simulink model "task3"  (R2023b)
settings: Solver=FixedStepDiscrete  StartTime=0.0  StopTime=10.0  FixedStep=5e-5  RelTol=1e-3
PreLoadFcn:
  | Simulink.defineIntEnumType('windowCommand', {'Off','Speed1','Speed2','Speed3'},[0,1,2,3])
settings Model: Creator=kz1nz0  LastModifiedBy=Zuzia

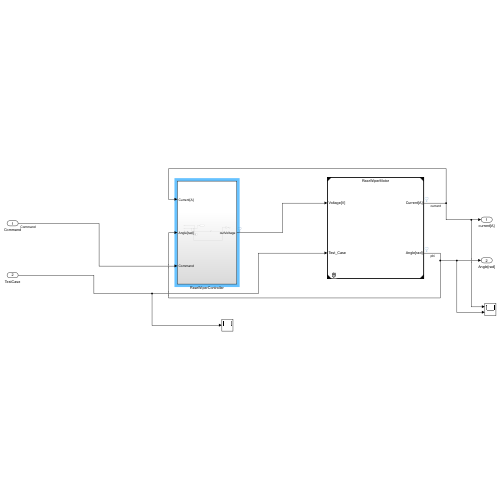
[thumbnail: Simulink's stored preview of the top-level diagram]
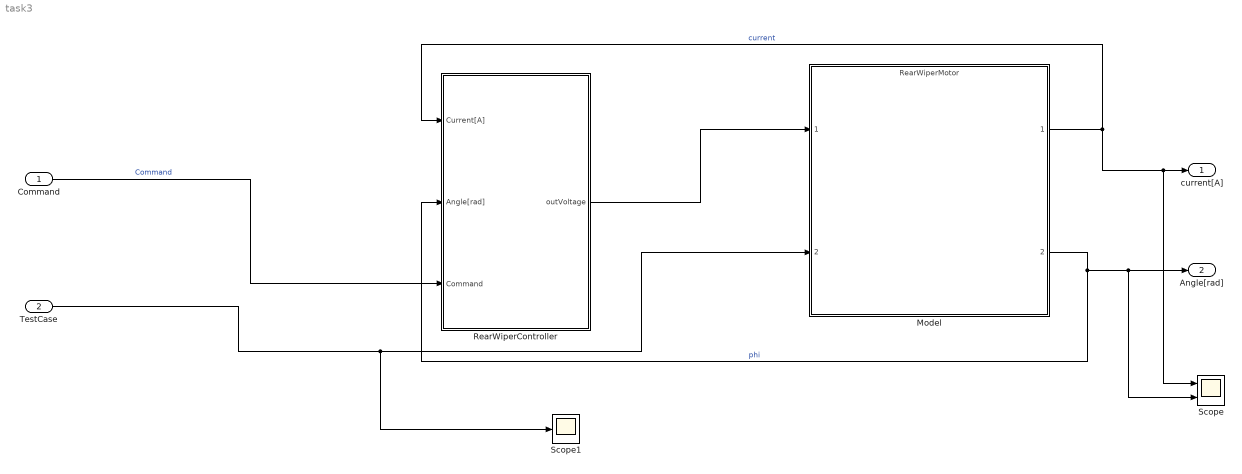
== system task3 ==
  Command : Inport  OutDataTypeStr=Enum: windowCommand
  TestCase : Inport  Port=2  OutDataTypeStr=int8
  Model : ModelReference  ModelNameDialog=RearWiperMotor.slxp  ModelReferenceVersion=19.15  CopyOfModelProtected=on
  RearWiperController : Subsystem
  Scope : Scope  NumInputPorts=2
  Scope1 : Scope
  current[A] : Outport
  Angle[rad] : Outport  Port=2
  wires:
  Command/1 -> RearWiperController/3(Command)  "Command"
  TestCase/1 -> Scope1/1, Model/2
  Model/1 -> Scope/1, current[A]/1, RearWiperController/1(Current[A])  "current"
  Model/2 -> RearWiperController/2(Angle[rad]), Scope/2, Angle[rad]/1  "phi"
  RearWiperController/1(outVoltage) -> Model/1

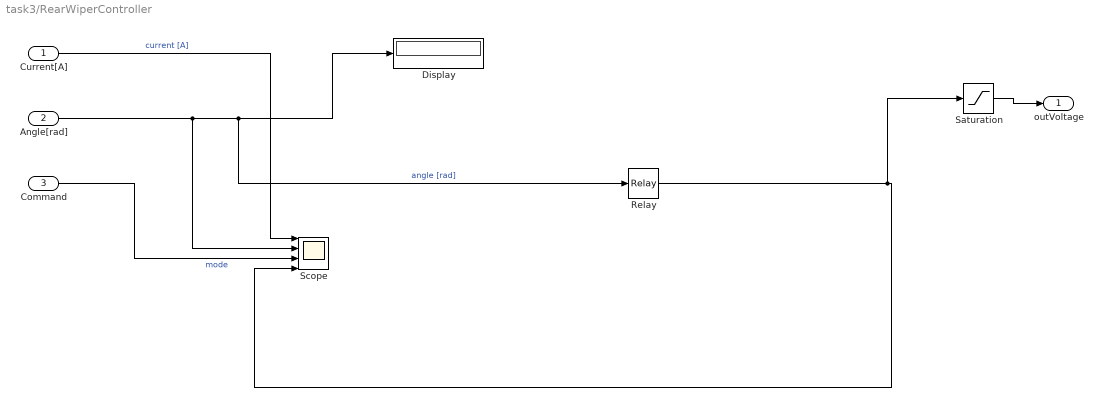
== system task3/RearWiperController ==
  Current[A] : Inport
  Angle[rad] : Inport  Port=2
  Command : Inport  Port=3  OutDataTypeStr=Enum: windowCommand
  Display : Display
  Relay : Relay  OnSwitchValue=2.7  OffSwitchValue=0  OnOutputValue=-5  OffOutputValue=5
  Saturation : Saturate  UpperLimit=12  LowerLimit=-12
  Scope : Scope  NumInputPorts=4
  outVoltage : Outport
  wires:
  Command/1 -> Scope/3  "mode"
  Angle[rad]/1 -> Scope/2, Relay/1, Display/1  "angle [rad]"
  Current[A]/1 -> Scope/1  "current [A]"
  Relay/1 -> Saturation/1, Scope/4
  Saturation/1 -> outVoltage/1
